simulink model "OBCSystem"  (R2025b)
settings: Solver=FixedStepAuto  StartTime=0.0  StopTime=100e-3  RelTol=1e-3  EnableMultiTasking=on
PreLoadFcn:
  | %% Load OBCSystem initialization parameters
  | initScriptPath = fullfile(fileparts(which('OBCSystem')), '..', 'SupportFiles', 'Scripts', 'OBCSystem_init.m');
  | if isfile(initScriptPath)
  |     evalin('base', fileread(initScriptPath));
  | else
  |     warning('OBCSystem:initNotFound', 'OBCSystem_init.m not found at: %s', initScriptPath);
  | end
InitFcn:
  | mode = str2double(get_param('OBCSystem/System/SimulationMode','value'));
  | enableLogging = str2double(get_param('OBCSystem/System/On-Board Charger/HIL/EnableHighResLogging','value'));
  | 
  | % If the charger runs on the FPGA AND high-resolution logging is enabled,
  | % uncomment interrupt setup. Comment otherwise
  | if ((mode == 2) && (enableLogging == 1))
  |     set_param('OBCSystem/Interrupt Setup','Commented','off');
  | else
  |     set_param('OBCSystem/Interrupt Setup','Commented','on');
  | end
  | 
  | % If DMA streaming is enambled and simulation time exceeds 30s, then throw an error
  | maxStopTime = 30;   % seconds
  | stopTimeStr = get_param(bdroot, 'StopTime');
  | stopTimeVal = str2double(stopTimeStr);
  | 
  | if enableLogging && stopTimeVal > maxStopTime
  |     error('DMA streaming is enabled, but StopTime = %.3f s exceeds the allowed %.3f s.', ...
  |           stopTimeVal, maxStopTime);
  | end
undefined symbols (not defined in the file): DAB, DAB_CCCV_Ki, DAB_CCCV_Kp, DAB_CCCV_Kt, DAB_Charging, DAB_CurrentReference, DAB_DCOffset, DAB_PhaseShift_LowerSat, DAB_PhaseShift_UpperSat, DAB_PhaseShiftInit, DAB_PhaseToDeg, DAB_PID_Kd, DAB_PID_Ki, DAB_PID_Kp, DAB_PID_LowerSat, DAB_PID_N, DAB_PID_UpperSat, Fourier_class, FPGA, FrameSize, getfullname, grid, Instr_EffGain, Instr_PinGain, Instr_PoutGain, Instr_pUtoDeg, Instr_RippleGain, Instr_SoCGain, IO334, Ki_current, Ki_voltage, Kp_current, Kp_voltage, MIL_or_HIL, OBC_template1, OpenLoopDuty, OpenLoopEnable, PCIe_RT, PFC_Current_Kb, PFC_Current_LowerSat, PFC_Current_UpperSat, PFC_Sat_DC_Lower, PFC_Sat_DC_Upper, PFC_Sat_iL_Lower, PFC_Sat_iL_Upper, PFC_Sat_Pwr_Lower, PFC_Sat_Pwr_Upper, PFC_Voltage_Kb, PFC_Voltage_LowerSat, PFC_Voltage_UpperSat, Rblock, Real, Time, totemPole, ts_CPU, ts_FPGA_clk, ts_FPGA_mdl, VectorSize
libraries: nesl_utility x27, fl_lib x24, speedgoatlib_hdlCoder_IO3xx x20, ee_lib x12, simulink x4, eeGeneralControl x4, slpidlib x3, pwm_cpulib x2, batteryecm_lib x2, slrealtimeloglib x2, pwm_fpgalib x2, speedgoatlib_interrupt x1
(part 4 of 4)

== system OBCSystem/System/On-Board Charger/HIL/Battery circuit/Temperature Sensor1 ==
  Temperature Sensor : fl_lib/Thermal/Thermal Sensors/Temperature Sensor  temperature_measure=foundation.enum.MeasurementReference.difference
  Thermal Reference : fl_lib/Thermal/Thermal Elements/Thermal Reference
  H : PMIOPort  Side=Left
  T : PMIOPort  Port=2  Side=Left
  connections:
  H/RConn1 -- Temperature Sensor/LConn1
  T/RConn1 -- Temperature Sensor/RConn2
  Temperature Sensor/RConn1 -- Thermal Reference/LConn1

== system OBCSystem/System/On-Board Charger/MIL/PWM/Gate Logic1 ==
  g : Inport
  Source Voltage Flag : Inport  Port=2
  Constant : Constant  Value=0  OutDataTypeStr=Inherit: Inherit via back propagation  SampleTime=ts_FPGA_mdl
  Constant1 : Constant  OutDataTypeStr=Inherit: Inherit via back propagation  SampleTime=ts_FPGA_mdl
  Mux : Mux
  Selector : Selector  InputPortWidth=4  IndexOptions=Index vector (dialog)  Indices=[2 1 4 3]  OutputSizes=1
  Switch : Switch  Criteria=u2 ~= 0  SaturateOnIntegerOverflow=off  InputSameDT=off
  Unit Delay : UnitDelay  SampleTime=-1
  PWM : Outport
  wires:
  Mux/1 -> Selector/1, Switch/1
  Selector/1 -> Switch/3
  Source Voltage Flag/1 -> Unit Delay/1
  Constant/1 -> Mux/3, Mux/1
  Constant1/1 -> Mux/4
  Switch/1 -> PWM/1
  g/1 -> Mux/2
  Unit Delay/1 -> Switch/2

== system OBCSystem/System/On-Board Charger/MIL/PWM/PWM Generation DAB  ==
  Configuration : Inport  Partition=on  PartitionDimension=1  PartitionWidth=16  PartitionOffset=0
  Runtime_CPU : Inport  Port=2  Partition=on  PartitionDimension=1  PartitionWidth=5  PartitionOffset=0
  Abstraction PWM Generation : pwm_fpgalib/Abstraction PWM Generation
      link override PWM FPGA Code Module/Carrier/HDL Counter: CountSampTime=1
      link override PWM FPGA Code Module/Carrier/HDL Counter/Count_reg: SampleTime=samptime
      settings: SourceProductName=PWM FPGA Library
  For Each : ForEach  DisableCoverage=on
  Mux : Mux
  Terminator : Terminator
  Zero : Constant  Value=zeros(1,3)  OutDataTypeStr=fixdt(1,32,31)  SampleTime=-1
  PWM Full Bridge : Outport  ConcatenationDimension=1
  wires:
  Abstraction PWM Generation/3 -> Terminator/1
  Runtime_CPU/1 -> Abstraction PWM Generation/2
  Zero/1 -> Abstraction PWM Generation/3
  Mux/1 -> PWM Full Bridge/1
  Configuration/1 -> Abstraction PWM Generation/1
  Abstraction PWM Generation/1 -> Mux/4, Mux/1
  Abstraction PWM Generation/2 -> Mux/3, Mux/2

== system OBCSystem/System/On-Board Charger/MIL/PWM/PWM Generation PFC ==
  PWM_Config : Inport
  PWM_Runtime : Inport  Port=2
  PWM_Enable : Inport  Port=3
  Disable_Gates : Constant  Value=[0]  OutDataTypeStr=boolean  SampleTime=-1
  For each subsystem: PWM Generation Abstraction : Subsystem
  Switch : Switch  Criteria=u2 ~= 0  SaturateOnIntegerOverflow=off  InputSameDT=off
  Terminator : Terminator
  Terminator1 : Terminator
  Zero : Constant  Value=zeros(1,3)  OutDataTypeStr=fixdt(1,32,31)  SampleTime=ts_FPGA_mdl
  1_Gate : Outport
  wires:
  Zero/1 -> For each subsystem: PWM Generation Abstraction/3(PWM_Runtime_FPGA)
  For each subsystem: PWM Generation Abstraction/1(pwm_a_o) -> Switch/1
  PWM_Enable/1 -> Switch/2
  Switch/1 -> 1_Gate/1
  Disable_Gates/1 -> Switch/3
  PWM_Runtime/1 -> For each subsystem: PWM Generation Abstraction/2(PWM_Runtime_CPU)
  PWM_Config/1 -> For each subsystem: PWM Generation Abstraction/1(PWM_Config)
  For each subsystem: PWM Generation Abstraction/2(pwm_b_o) -> Terminator/1
  For each subsystem: PWM Generation Abstraction/3(pwm_c_o) -> Terminator1/1

== system OBCSystem/System/On-Board Charger/MIL/Simscape/Temperature Sensor ==
  Temperature Sensor : fl_lib/Thermal/Thermal Sensors/Temperature Sensor  temperature_measure=foundation.enum.MeasurementReference.difference
  Thermal Reference : fl_lib/Thermal/Thermal Elements/Thermal Reference
  H : PMIOPort  Side=Left
  T : PMIOPort  Port=2  Side=Left
  connections:
  H/RConn1 -- Temperature Sensor/LConn1
  T/RConn1 -- Temperature Sensor/RConn2
  Temperature Sensor/RConn1 -- Thermal Reference/LConn1

== system OBCSystem/System/On-Board Charger/MIL/PWM/PWM Generation PFC/For each subsystem: PWM Generation Abstraction ==
  PWM_Config : Inport  Partition=on  PartitionDimension=1  PartitionWidth=16  PartitionOffset=0
  PWM_Runtime_CPU : Inport  Port=2  Partition=on  PartitionDimension=1  PartitionWidth=5  PartitionOffset=0
  PWM_Runtime_FPGA : Inport  Port=3
  Abstraction PWM Generation : pwm_fpgalib/Abstraction PWM Generation
      settings: SourceProductName=PWM FPGA Library
  For Each : ForEach  DisableCoverage=on
  pwm_a_o : Outport  ConcatenationDimension=1
  pwm_b_o : Outport  Port=2  ConcatenationDimension=1
  pwm_c_o : Outport  Port=3  ConcatenationDimension=1
  wires:
  PWM_Config/1 -> Abstraction PWM Generation/1
  PWM_Runtime_CPU/1 -> Abstraction PWM Generation/2
  Abstraction PWM Generation/1 -> pwm_a_o/1
  Abstraction PWM Generation/3 -> pwm_c_o/1
  Abstraction PWM Generation/2 -> pwm_b_o/1
  PWM_Runtime_FPGA/1 -> Abstraction PWM Generation/3
